simulink model "three_phase_inv"  (R2021a)
settings: Solver=VariableStepAuto  StartTime=0.0  StopTime=10.0  RelTol=1e-3
libraries: spsIGBTLib x6, spsSeriesRLCBranchLib x3, spsTriangleGeneratorLib x3, spsVoltageMeasurementLib x2, spsCurrentMeasurementLib x1, spsDCVoltageSourceLib x1, spspowerguiLib x1
settings Model: Creator=HP  LastModifiedBy=mansi
settings SolverCC: AlgebraicLoopSolver=TrustRegion
settings DebuggingCC: SFMachineParentedDataDiag=warning

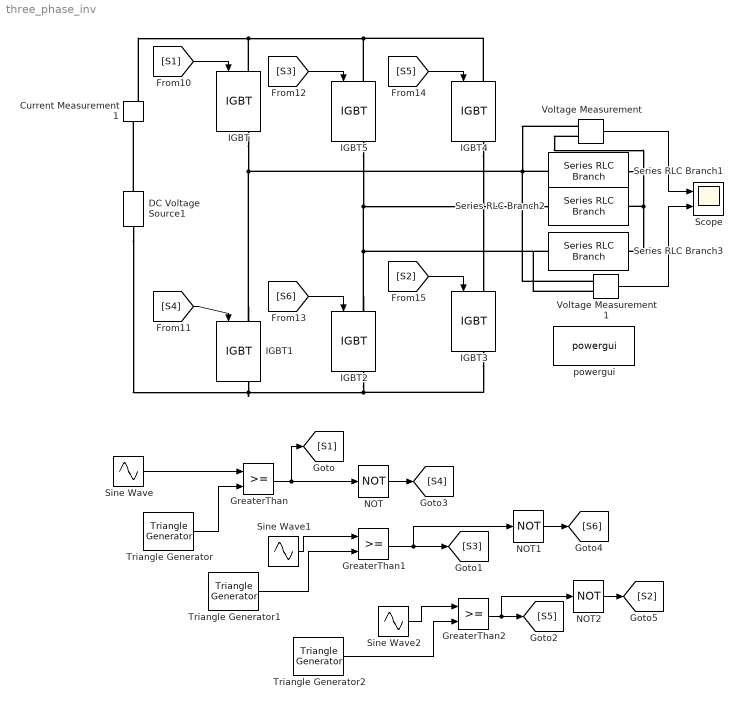
== system three_phase_inv ==
  Current Measurement1 : spsCurrentMeasurementLib/Current Measurement  PhasorSimulation=off  OutputType=Complex  PSBequivalent=0
  DC Voltage Source1 : spsDCVoltageSourceLib/DC Voltage Source  Amplitude=800  Measurements=None
  GreaterThan : RelationalOperator  OutDataTypeStr=boolean  RndMeth=Simplest
  GreaterThan1 : RelationalOperator  OutDataTypeStr=boolean  RndMeth=Simplest
  GreaterThan2 : RelationalOperator  OutDataTypeStr=boolean  RndMeth=Simplest
  IGBT{,1..5} (6 alike) : spsIGBTLib/IGBT  Ron=20e-3  Lon=0  Vf=0.7  Tf=1e-6  Tt=2e-6  IC=0  Rs=1e5  Cs=inf  Measurements=on
  NOT : Logic  Operator=NOT  IconShape=distinctive  AllPortsSameDT=off  OutDataTypeStr=boolean
  NOT1 : Logic  Operator=NOT  IconShape=distinctive  AllPortsSameDT=off  OutDataTypeStr=boolean
  NOT2 : Logic  Operator=NOT  IconShape=distinctive  AllPortsSameDT=off  OutDataTypeStr=boolean
  Scope : Scope  NumInputPorts=2
  Series RLC Branch1 : spsSeriesRLCBranchLib/Series RLC Branch  LConnTagsString=__new0  RConnTagsString=__new0  BranchType=RL  Resistance=40  Inductance=20e-3  SetiL0=off  InitialCurrent=0  Capacitance=1e-6  Setx0=off  InitialVoltage=0  Measurements=None
  Series RLC Branch2 : spsSeriesRLCBranchLib/Series RLC Branch  LConnTagsString=__new0  RConnTagsString=__new0  BranchType=RL  Resistance=40  Inductance=20e-3  SetiL0=off  InitialCurrent=0  Capacitance=1e-6  Setx0=off  InitialVoltage=0  Measurements=None
  Series RLC Branch3 : spsSeriesRLCBranchLib/Series RLC Branch  LConnTagsString=__new0  RConnTagsString=__new0  BranchType=RL  Resistance=40  Inductance=20e-3  SetiL0=off  InitialCurrent=0  Capacitance=1e-6  Setx0=off  InitialVoltage=0  Measurements=None
  Sine Wave : Sin  Frequency=314  SampleTime=0
  Sine Wave1 : Sin  Frequency=314  Phase=-2*pi/3  SampleTime=0
  Sine Wave2 : Sin  Frequency=314  Phase=2*pi/3  SampleTime=0
  Triangle Generator : spsTriangleGeneratorLib/Triangle Generator  Freq=15e3  Phase=90  Ts=0
  Triangle Generator1 : spsTriangleGeneratorLib/Triangle Generator  Freq=15e3  Phase=90  Ts=0
  Triangle Generator2 : spsTriangleGeneratorLib/Triangle Generator  Freq=15e3  Phase=90  Ts=0
  Voltage Measurement : spsVoltageMeasurementLib/Voltage Measurement  PhasorSimulation=off  OutputType=Complex  PSBequivalent=0
  Voltage Measurement1 : spsVoltageMeasurementLib/Voltage Measurement  PhasorSimulation=off  OutputType=Complex  PSBequivalent=0
  powergui : spspowerguiLib/powergui  Priority=1  SimulationMode=Discrete  SampleTime=1e-7  frequency=60  Iterations=50  frequencyindice=60  Pbase=100e6  ErrMax=1e-4  UnitsV=kV  UnitsW=MW  buscounter=0  FunctionMessages=off  echomessages=off  EnableUseOfTLC=off  CurrentSourceSwitches=off  DisableSnubberDevices=off  DisableRonSwitches=off  DisableVfSwitches=off  DisplayEquations=off  AutomaticDiscreteSolvers=off  SolverType=Tustin/Backward Euler (TBE)  Interpol=off  ExternalGateDelay=off  methode=off  Ts=100  x0status=blocks  SPID=on  SwTol=0  HookPort=off  NonlinearTolerance=1e-4  nMaxIteration=100  ContinueOnMaxIteration=off  RestoreLinks=warning  ResistiveCurrentMeasurement=off  Frange=[0:2:500]  Ylog=off  Xlog=on  ShowGrid=off  save=off  variable=ZData  structure=0  ZoomFFT=off  StartTime=0.0  cycles=1  DisplayStyle=1  fundamental=60  FreqAxis=off  MaxFrequency=1000  frequencyindicesteady=1  RmsSteady=1  display=off
  wires:
  [S2] -> IGBT3/1
  [S5] -> IGBT4/1
  [S6] -> IGBT2/1
  [S4] -> IGBT1/1
  [S3] -> IGBT5/1
  [S1] -> IGBT/1
  GreaterThan/1 -> NOT/1, [S1]
  GreaterThan2/1 -> [S5], NOT2/1
  GreaterThan1/1 -> [S3], NOT1/1
  NOT/1 -> [S4]
  NOT1/1 -> [S6]
  Voltage Measurement/1 -> Scope/1
  Voltage Measurement1/1 -> Scope/2
  NOT2/1 -> [S2]
  Sine Wave1/1 -> GreaterThan1/1
  Triangle Generator2/1 -> GreaterThan2/2
  Triangle Generator1/1 -> GreaterThan1/2
  Sine Wave2/1 -> GreaterThan2/1
  Triangle Generator/1 -> GreaterThan/2
  Sine Wave/1 -> GreaterThan/1
  connections:
  IGBT5/RConn1 -- IGBT2/LConn1 -- Voltage Measurement1/LConn2 -- Series RLC Branch3/LConn1 -- Series RLC Branch2/LConn1
  Series RLC Branch1/RConn1 -- Series RLC Branch3/RConn1 -- Series RLC Branch2/RConn1 -- Voltage Measurement/LConn2
  Current Measurement1/RConn1 -- IGBT/LConn1 -- IGBT4/LConn1 -- IGBT5/LConn1
  Series RLC Branch1/LConn1 -- IGBT1/LConn1 -- IGBT/RConn1 -- Voltage Measurement1/LConn1 -- Voltage Measurement/LConn1
  DC Voltage Source1/LConn1 -- IGBT1/RConn1 -- IGBT3/RConn1 -- IGBT2/RConn1
  DC Voltage Source1/RConn1 -- Current Measurement1/LConn1
  IGBT4/RConn1 -- IGBT3/LConn1
